simulink model "RC_Circuit"  (R2020a)
settings: Solver=VariableStepAuto  StartTime=0.0  StopTime=10.0  RelTol=1e-3
values from neighbouring files (symbols this model uses):
  C = 10e-6    (= 1e-05)    [startup.m]
  R = 10    [startup.m]
libraries: simulink x2
settings Model: Creator=Viraj  LastModifiedBy=Viraj

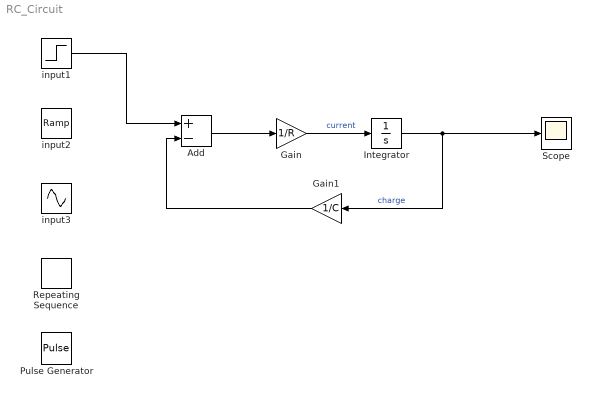
== system RC_Circuit ==
  Add : Sum  Inputs=+-
  Gain : Gain  Gain=1/R
  Gain1 : Gain  Gain=1/C
  Integrator : Integrator
  Pulse Generator : DiscretePulseGenerator  PulseType=Time based  Period=10  PulseWidth=5
  Repeating Sequence : simulink/Sources/Repeating Sequence  rep_seq_t=[0 2]  rep_seq_y=[0 2]
  Scope : Scope
  input1 : Step  SampleTime=0
  input2 : simulink/Sources/Ramp  slope=1  start=0  InitialOutput=0
  input3 : Sin  SampleTime=0
  wires:
  Gain/1 -> Integrator/1  "current"
  Integrator/1 -> Scope/1, Gain1/1  "charge"
  Add/1 -> Gain/1
  Gain1/1 -> Add/2
  input1/1 -> Add/1
